simulink model "Testbed_v3"  (R2020a)
settings: Solver=ode23tb  StartTime=0.0  StopTime=20  MaxStep=0.066666666666666671  RelTol=1e-4  EnableMultiTasking=on
undefined symbols (not defined in the file): D11, Delta
libraries: powerlib x95, dspnetwork x75, dspstat3 x52, eePMU x16
(part 2 of 2)

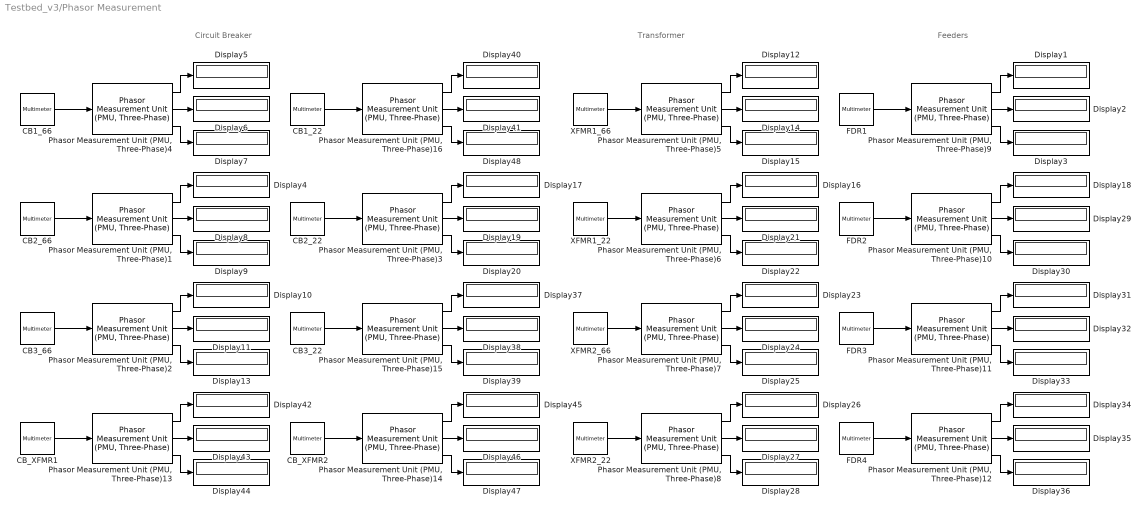
== system Testbed_v3/Phasor Measurement ==
  note: Circuit Breaker
  note: Transformer
  note: Feeders
  CB1_22 : powerlib/Measurements/Multimeter  PhasorSimulation=off  OutputType=Complex  sel=[13 14 15]  L=198  Gain=[1 1 1]  yselected={'Ub: CB1_22KV/Breaker A','Ub: CB1_22KV/Breaker B','Ub: CB1_22KV/Breaker C'};  PSBOutputType=1  PSBequivalent=0  AxesSetting=[0,0.1,-100,100]  Display=0  SavedBlockNames=-11
  CB1_66 : powerlib/Measurements/Multimeter  PhasorSimulation=off  OutputType=Complex  sel=[16 17 18]  L=198  Gain=[1 1 1]  yselected={'Ub: CB1_66KV/Breaker A','Ub: CB1_66KV/Breaker B','Ub: CB1_66KV/Breaker C'};  PSBOutputType=1  PSBequivalent=0  AxesSetting=[0,0.1,-100,100]  Display=0  SavedBlockNames=-11
  CB2_22 : powerlib/Measurements/Multimeter  PhasorSimulation=off  OutputType=Complex  sel=[19 20 21]  L=198  Gain=[1 1 1]  yselected={'Ub: CB2_22KV/Breaker A','Ub: CB2_22KV/Breaker B','Ub: CB2_22KV/Breaker C'};  PSBOutputType=1  PSBequivalent=0  AxesSetting=[0,0.1,-100,100]  Display=0  SavedBlockNames=-11
  CB2_66 : powerlib/Measurements/Multimeter  PhasorSimulation=off  OutputType=Complex  sel=[22 23 24]  L=198  Gain=[1 1 1]  yselected={'Ub: CB2_66KV/Breaker A','Ub: CB2_66KV/Breaker B','Ub: CB2_66KV/Breaker C'};  PSBOutputType=1  PSBequivalent=0  AxesSetting=[0,0.1,-100,100]  Display=0  SavedBlockNames=-11
  CB3_22 : powerlib/Measurements/Multimeter  PhasorSimulation=off  OutputType=Complex  sel=[25 26 27]  L=198  Gain=[1 1 1]  yselected={'Ub: CB3_22KV/Breaker A','Ub: CB3_22KV/Breaker B','Ub: CB3_22KV/Breaker C'};  PSBOutputType=1  PSBequivalent=0  AxesSetting=[0,0.1,-100,100]  Display=0  SavedBlockNames=-11
  CB3_66 : powerlib/Measurements/Multimeter  PhasorSimulation=off  OutputType=Complex  sel=[28 29 30]  L=198  Gain=[1 1 1]  yselected={'Ub: CB3_66KV/Breaker A','Ub: CB3_66KV/Breaker B','Ub: CB3_66KV/Breaker C'};  PSBOutputType=1  PSBequivalent=0  AxesSetting=[0,0.1,-100,100]  Display=0  SavedBlockNames=-11
  CB_XFMR1 : powerlib/Measurements/Multimeter  PhasorSimulation=off  OutputType=Complex  sel=[43 44 45]  L=198  Gain=[1 1 1]  yselected={'Ub: CB_XFMR1/Breaker A','Ub: CB_XFMR1/Breaker B','Ub: CB_XFMR1/Breaker C'};  PSBOutputType=1  PSBequivalent=0  AxesSetting=[0,0.1,-100,100]  Display=0  SavedBlockNames=-11
  CB_XFMR2 : powerlib/Measurements/Multimeter  PhasorSimulation=off  OutputType=Complex  sel=[46 47 48]  L=198  Gain=[1 1 1]  yselected={'Ub: CB_XFMR2/Breaker A','Ub: CB_XFMR2/Breaker B','Ub: CB_XFMR2/Breaker C'};  PSBOutputType=1  PSBequivalent=0  AxesSetting=[0,0.1,-100,100]  Display=0  SavedBlockNames=-11
  Display{1..48} (48 alike) : Display
  FDR1 : powerlib/Measurements/Multimeter  PhasorSimulation=off  OutputType=Complex  sel=[31 32 33]  L=198  Gain=[1 1 1]  yselected={'Ub: CB_FDR1/Breaker A','Ub: CB_FDR1/Breaker B','Ub: CB_FDR1/Breaker C'};  PSBOutputType=1  PSBequivalent=0  AxesSetting=[0,0.1,-100,100]  Display=0  SavedBlockNames=-11
  FDR2 : powerlib/Measurements/Multimeter  PhasorSimulation=off  OutputType=Complex  sel=[34 35 36]  L=198  Gain=[1 1 1]  yselected={'Ub: CB_FDR2/Breaker A','Ub: CB_FDR2/Breaker B','Ub: CB_FDR2/Breaker C'};  PSBOutputType=1  PSBequivalent=0  AxesSetting=[0,0.1,-100,100]  Display=0  SavedBlockNames=-11
  FDR3 : powerlib/Measurements/Multimeter  PhasorSimulation=off  OutputType=Complex  sel=[37 38 39]  L=198  Gain=[1 1 1]  yselected={'Ub: CB_FDR3/Breaker A','Ub: CB_FDR3/Breaker B','Ub: CB_FDR3/Breaker C'};  PSBOutputType=1  PSBequivalent=0  AxesSetting=[0,0.1,-100,100]  Display=0  SavedBlockNames=-11
  FDR4 : powerlib/Measurements/Multimeter  PhasorSimulation=off  OutputType=Complex  sel=[40 41 42]  L=198  Gain=[1 1 1]  yselected={'Ub: CB_FDR4/Breaker A','Ub: CB_FDR4/Breaker B','Ub: CB_FDR4/Breaker C'};  PSBOutputType=1  PSBequivalent=0  AxesSetting=[0,0.1,-100,100]  Display=0  SavedBlockNames=-11
  Phasor Measurement Unit (PMU, Three-Phase){1..16} (16 alike) : eePMU/Phasor Measurement Unit (PMU, Three-Phase)  frequency=50  Nsr=64  k=1
      settings: SourceProductBaseCode=PS
  XFMR1_22 : powerlib/Measurements/Multimeter  PhasorSimulation=off  OutputType=Complex  sel=[82 82 82]  L=198  Gain=[1 1 1]  yselected={'Uab_w2: Three-Phase Transformer 1 (Two Windings)','Uab_w2: Three-Phase Transformer 1 (Two Windings)','Uab_w2: Three-Phase Transformer 1 (Two Windings)'};  PSBOutputType=1  PSBequivalent=0  AxesSetting=[0,0.1,-100,100]  Display=0  SavedBlockNames=-11
  XFMR1_66 : powerlib/Measurements/Multimeter  PhasorSimulation=off  OutputType=Complex  sel=[79 79 79]  L=198  Gain=[1 1 1]  yselected={'Uag_w1: Three-Phase Transformer 1 (Two Windings)','Uag_w1: Three-Phase Transformer 1 (Two Windings)','Uag_w1: Three-Phase Transformer 1 (Two Windings)'};  PSBOutputType=1  PSBequivalent=0  AxesSetting=[0,0.1,-100,100]  Display=0  SavedBlockNames=-11
  XFMR2_22 : powerlib/Measurements/Multimeter  PhasorSimulation=off  OutputType=Complex  sel=[88 88 88]  L=198  Gain=[1 1 1]  yselected={'Uab_w2: Three-Phase Transformer 2 (Two Windings)','Uab_w2: Three-Phase Transformer 2 (Two Windings)','Uab_w2: Three-Phase Transformer 2 (Two Windings)'};  PSBOutputType=1  PSBequivalent=0  AxesSetting=[0,0.1,-100,100]  Display=0  SavedBlockNames=-11
  XFMR2_66 : powerlib/Measurements/Multimeter  PhasorSimulation=off  OutputType=Complex  sel=[85 85 85]  L=198  Gain=[1 1 1]  yselected={'Uag_w1: Three-Phase Transformer 2 (Two Windings)','Uag_w1: Three-Phase Transformer 2 (Two Windings)','Uag_w1: Three-Phase Transformer 2 (Two Windings)'};  PSBOutputType=1  PSBequivalent=0  AxesSetting=[0,0.1,-100,100]  Display=0  SavedBlockNames=-11
  wires:
  CB1_66/1 -> "Phasor Measurement Unit (PMU, Three-Phase)4"/1
  CB2_66/1 -> "Phasor Measurement Unit (PMU, Three-Phase)1"/1
  CB3_66/1 -> "Phasor Measurement Unit (PMU, Three-Phase)2"/1
  XFMR1_22/1 -> "Phasor Measurement Unit (PMU, Three-Phase)6"/1
  XFMR2_66/1 -> "Phasor Measurement Unit (PMU, Three-Phase)7"/1
  CB2_22/1 -> "Phasor Measurement Unit (PMU, Three-Phase)3"/1
  FDR1/1 -> "Phasor Measurement Unit (PMU, Three-Phase)9"/1
  FDR2/1 -> "Phasor Measurement Unit (PMU, Three-Phase)10"/1
  FDR3/1 -> "Phasor Measurement Unit (PMU, Three-Phase)11"/1
  FDR4/1 -> "Phasor Measurement Unit (PMU, Three-Phase)12"/1
  XFMR1_66/1 -> "Phasor Measurement Unit (PMU, Three-Phase)5"/1
  XFMR2_22/1 -> "Phasor Measurement Unit (PMU, Three-Phase)8"/1
  "Phasor Measurement Unit (PMU, Three-Phase)4"/1 -> Display5/1
  "Phasor Measurement Unit (PMU, Three-Phase)4"/2 -> Display6/1
  "Phasor Measurement Unit (PMU, Three-Phase)4"/3 -> Display7/1
  "Phasor Measurement Unit (PMU, Three-Phase)1"/2 -> Display8/1
  "Phasor Measurement Unit (PMU, Three-Phase)1"/3 -> Display9/1
  "Phasor Measurement Unit (PMU, Three-Phase)1"/1 -> Display4/1
  "Phasor Measurement Unit (PMU, Three-Phase)2"/2 -> Display11/1
  "Phasor Measurement Unit (PMU, Three-Phase)2"/3 -> Display13/1
  "Phasor Measurement Unit (PMU, Three-Phase)2"/1 -> Display10/1
  "Phasor Measurement Unit (PMU, Three-Phase)3"/2 -> Display19/1
  "Phasor Measurement Unit (PMU, Three-Phase)3"/3 -> Display20/1
  "Phasor Measurement Unit (PMU, Three-Phase)3"/1 -> Display17/1
  "Phasor Measurement Unit (PMU, Three-Phase)5"/2 -> Display14/1
  "Phasor Measurement Unit (PMU, Three-Phase)5"/3 -> Display15/1
  "Phasor Measurement Unit (PMU, Three-Phase)5"/1 -> Display12/1
  "Phasor Measurement Unit (PMU, Three-Phase)6"/2 -> Display21/1
  "Phasor Measurement Unit (PMU, Three-Phase)6"/3 -> Display22/1
  "Phasor Measurement Unit (PMU, Three-Phase)6"/1 -> Display16/1
  "Phasor Measurement Unit (PMU, Three-Phase)7"/2 -> Display24/1
  "Phasor Measurement Unit (PMU, Three-Phase)7"/3 -> Display25/1
  "Phasor Measurement Unit (PMU, Three-Phase)7"/1 -> Display23/1
  "Phasor Measurement Unit (PMU, Three-Phase)8"/2 -> Display27/1
  "Phasor Measurement Unit (PMU, Three-Phase)8"/3 -> Display28/1
  "Phasor Measurement Unit (PMU, Three-Phase)8"/1 -> Display26/1
  "Phasor Measurement Unit (PMU, Three-Phase)9"/2 -> Display2/1
  "Phasor Measurement Unit (PMU, Three-Phase)9"/3 -> Display3/1
  "Phasor Measurement Unit (PMU, Three-Phase)9"/1 -> Display1/1
  "Phasor Measurement Unit (PMU, Three-Phase)10"/2 -> Display29/1
  "Phasor Measurement Unit (PMU, Three-Phase)10"/3 -> Display30/1
  "Phasor Measurement Unit (PMU, Three-Phase)10"/1 -> Display18/1
  "Phasor Measurement Unit (PMU, Three-Phase)11"/2 -> Display32/1
  "Phasor Measurement Unit (PMU, Three-Phase)11"/3 -> Display33/1
  "Phasor Measurement Unit (PMU, Three-Phase)11"/1 -> Display31/1
  "Phasor Measurement Unit (PMU, Three-Phase)12"/2 -> Display35/1
  "Phasor Measurement Unit (PMU, Three-Phase)12"/3 -> Display36/1
  "Phasor Measurement Unit (PMU, Three-Phase)12"/1 -> Display34/1
  "Phasor Measurement Unit (PMU, Three-Phase)13"/3 -> Display44/1
  "Phasor Measurement Unit (PMU, Three-Phase)13"/2 -> Display43/1
  "Phasor Measurement Unit (PMU, Three-Phase)13"/1 -> Display42/1
  CB_XFMR1/1 -> "Phasor Measurement Unit (PMU, Three-Phase)13"/1
  "Phasor Measurement Unit (PMU, Three-Phase)14"/3 -> Display47/1
  "Phasor Measurement Unit (PMU, Three-Phase)14"/2 -> Display46/1
  "Phasor Measurement Unit (PMU, Three-Phase)14"/1 -> Display45/1
  CB_XFMR2/1 -> "Phasor Measurement Unit (PMU, Three-Phase)14"/1
  CB3_22/1 -> "Phasor Measurement Unit (PMU, Three-Phase)15"/1
  "Phasor Measurement Unit (PMU, Three-Phase)15"/3 -> Display39/1
  "Phasor Measurement Unit (PMU, Three-Phase)15"/1 -> Display37/1
  "Phasor Measurement Unit (PMU, Three-Phase)15"/2 -> Display38/1
  CB1_22/1 -> "Phasor Measurement Unit (PMU, Three-Phase)16"/1
  "Phasor Measurement Unit (PMU, Three-Phase)16"/3 -> Display48/1
  "Phasor Measurement Unit (PMU, Three-Phase)16"/1 -> Display40/1
  "Phasor Measurement Unit (PMU, Three-Phase)16"/2 -> Display41/1

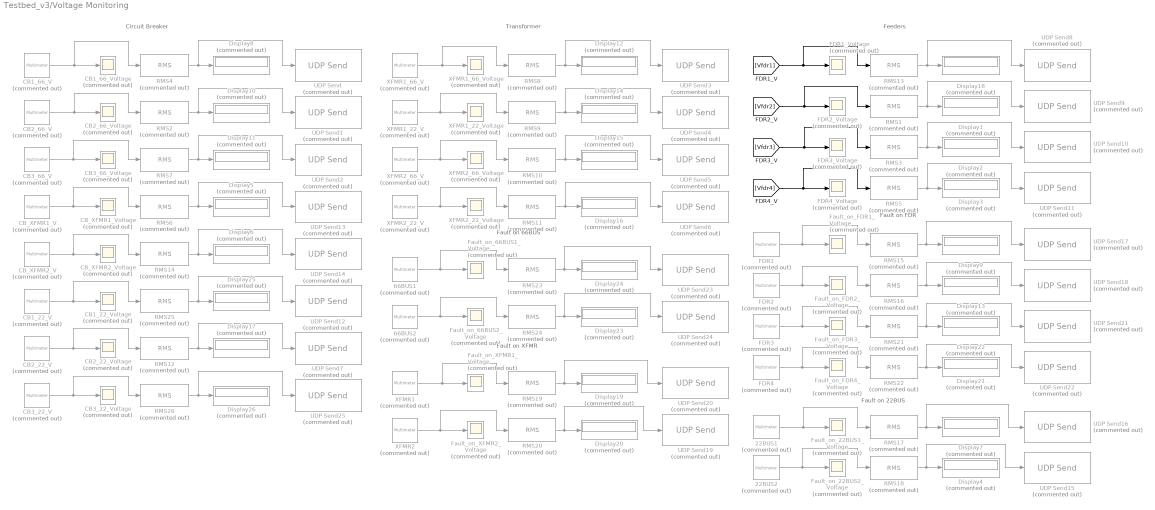
== system Testbed_v3/Voltage Monitoring ==
  note: Circuit Breaker
  note: Transformer
  note: Feeders
  note: Fault on XFMR
  note: Fault on 66BUS
  note: Fault on FDR
  note: Fault on 22BUS
  22BUS1 : powerlib/Measurements/Multimeter  Commented=on  PhasorSimulation=off  OutputType=Complex  sel=[49 50 51]  L=198  Gain=[1 1 1]  yselected={'Ub: Fault_22bus1/Fault A','Ub: Fault_22bus1/Fault B','Ub: Fault_22bus1/Fault C'};  PSBOutputType=1  PSBequivalent=0  AxesSetting=[0,0.1,-100,100]  Display=0  SavedBlockNames=-11
  22BUS2 : powerlib/Measurements/Multimeter  Commented=on  PhasorSimulation=off  OutputType=Complex  sel=[52 53 54]  L=198  Gain=[1 1 1]  yselected={'Ub: Fault_22bus2/Fault A','Ub: Fault_22bus2/Fault B','Ub: Fault_22bus2/Fault C'};  PSBOutputType=1  PSBequivalent=0  AxesSetting=[0,0.1,-100,100]  Display=0  SavedBlockNames=-11
  66BUS1 : powerlib/Measurements/Multimeter  Commented=on  PhasorSimulation=off  OutputType=Complex  sel=[55 56 57]  L=198  Gain=[1 1 1]  yselected={'Ub: Fault_66bus1/Fault A','Ub: Fault_66bus1/Fault B','Ub: Fault_66bus1/Fault C'};  PSBOutputType=1  PSBequivalent=0  AxesSetting=[0,0.1,-100,100]  Display=0  SavedBlockNames=-11
  66BUS2 : powerlib/Measurements/Multimeter  Commented=on  PhasorSimulation=off  OutputType=Complex  sel=[58 59 60]  L=198  Gain=[1 1 1]  yselected={'Ub: Fault_66bus2/Fault A','Ub: Fault_66bus2/Fault B','Ub: Fault_66bus2/Fault C'};  PSBOutputType=1  PSBequivalent=0  AxesSetting=[0,0.1,-100,100]  Display=0  SavedBlockNames=-11
  CB1_22_V : powerlib/Measurements/Multimeter  Commented=on  PhasorSimulation=off  OutputType=Complex  sel=[13 14 15]  L=198  Gain=[1 1 1]  yselected={'Ub: CB1_22KV/Breaker A','Ub: CB1_22KV/Breaker B','Ub: CB1_22KV/Breaker C'};  PSBOutputType=1  PSBequivalent=0  AxesSetting=[0,0.1,-100,100]  Display=0  SavedBlockNames=-11
  CB1_22_Voltage : Scope  Commented=on
  CB1_66_V : powerlib/Measurements/Multimeter  Commented=on  PhasorSimulation=off  OutputType=Complex  sel=[16 17 18]  L=198  Gain=[1 1 1]  yselected={'Ub: CB1_66KV/Breaker A','Ub: CB1_66KV/Breaker B','Ub: CB1_66KV/Breaker C'};  PSBOutputType=1  PSBequivalent=0  AxesSetting=[0,0.1,-100,100]  Display=0  SavedBlockNames=-11
  CB1_66_Voltage : Scope  Commented=on
  CB2_22_V : powerlib/Measurements/Multimeter  Commented=on  PhasorSimulation=off  OutputType=Complex  sel=[19 20 21]  L=198  Gain=[1 1 1]  yselected={'Ub: CB2_22KV/Breaker A','Ub: CB2_22KV/Breaker B','Ub: CB2_22KV/Breaker C'};  PSBOutputType=1  PSBequivalent=0  AxesSetting=[0,0.1,-100,100]  Display=0  SavedBlockNames=-11
  CB2_22_Voltage : Scope  Commented=on
  CB2_66_V : powerlib/Measurements/Multimeter  Commented=on  PhasorSimulation=off  OutputType=Complex  sel=[22 23 24]  L=198  Gain=[1 1 1]  yselected={'Ub: CB2_66KV/Breaker A','Ub: CB2_66KV/Breaker B','Ub: CB2_66KV/Breaker C'};  PSBOutputType=1  PSBequivalent=0  AxesSetting=[0,0.1,-100,100]  Display=0  SavedBlockNames=-11
  CB2_66_Voltage : Scope  Commented=on
  CB3_22_V : powerlib/Measurements/Multimeter  Commented=on  PhasorSimulation=off  OutputType=Complex  sel=[25 26 27]  L=198  Gain=[1 1 1]  yselected={'Ub: CB3_22KV/Breaker A','Ub: CB3_22KV/Breaker B','Ub: CB3_22KV/Breaker C'};  PSBOutputType=1  PSBequivalent=0  AxesSetting=[0,0.1,-100,100]  Display=0  SavedBlockNames=-11
  CB3_22_Voltage : Scope  Commented=on
  CB3_66_V : powerlib/Measurements/Multimeter  Commented=on  PhasorSimulation=off  OutputType=Complex  sel=[28 29 30]  L=198  Gain=[1 1 1]  yselected={'Ub: CB3_66KV/Breaker A','Ub: CB3_66KV/Breaker B','Ub: CB3_66KV/Breaker C'};  PSBOutputType=1  PSBequivalent=0  AxesSetting=[0,0.1,-100,100]  Display=0  SavedBlockNames=-11
  CB3_66_Voltage : Scope  Commented=on
  CB_XFMR1_V : powerlib/Measurements/Multimeter  Commented=on  PhasorSimulation=off  OutputType=Complex  sel=[43 44 45]  L=198  Gain=[1 1 1]  yselected={'Ub: CB_XFMR1/Breaker A','Ub: CB_XFMR1/Breaker B','Ub: CB_XFMR1/Breaker C'};  PSBOutputType=1  PSBequivalent=0  AxesSetting=[0,0.1,-100,100]  Display=0  SavedBlockNames=-11
  CB_XFMR1_Voltage : Scope  Commented=on
  CB_XFMR2_V : powerlib/Measurements/Multimeter  Commented=on  PhasorSimulation=off  OutputType=Complex  sel=[46 47 48]  L=198  Gain=[1 1 1]  yselected={'Ub: CB_XFMR2/Breaker A','Ub: CB_XFMR2/Breaker B','Ub: CB_XFMR2/Breaker C'};  PSBOutputType=1  PSBequivalent=0  AxesSetting=[0,0.1,-100,100]  Display=0  SavedBlockNames=-11
  CB_XFMR2_Voltage : Scope  Commented=on
  Display{1..26} (26 alike) : Display  Commented=on
  FDR1 : powerlib/Measurements/Multimeter  Commented=on  PhasorSimulation=off  OutputType=Complex  sel=[61 62 63]  L=198  Gain=[1 1 1]  yselected={'Ub: Fault_FDR1/Fault A','Ub: Fault_FDR1/Fault B','Ub: Fault_FDR1/Fault C'};  PSBOutputType=1  PSBequivalent=0  AxesSetting=[0,0.1,-100,100]  Display=0  SavedBlockNames=-11
  FDR1_Voltage : Scope  Commented=on
  FDR2 : powerlib/Measurements/Multimeter  Commented=on  PhasorSimulation=off  OutputType=Complex  sel=[64 65 66]  L=198  Gain=[1 1 1]  yselected={'Ub: Fault_FDR2/Fault A','Ub: Fault_FDR2/Fault B','Ub: Fault_FDR2/Fault C'};  PSBOutputType=1  PSBequivalent=0  AxesSetting=[0,0.1,-100,100]  Display=0  SavedBlockNames=-11
  FDR2_Voltage : Scope  Commented=on
  FDR3 : powerlib/Measurements/Multimeter  Commented=on  PhasorSimulation=off  OutputType=Complex  sel=[67 68 69]  L=198  Gain=[1 1 1]  yselected={'Ub: Fault_FDR3/Fault A','Ub: Fault_FDR3/Fault B','Ub: Fault_FDR3/Fault C'};  PSBOutputType=1  PSBequivalent=0  AxesSetting=[0,0.1,-100,100]  Display=0  SavedBlockNames=-11
  FDR3_Voltage : Scope  Commented=on
  FDR4 : powerlib/Measurements/Multimeter  Commented=on  PhasorSimulation=off  OutputType=Complex  sel=[70 71 72]  L=198  Gain=[1 1 1]  yselected={'Ub: Fault_FDR4/Fault A','Ub: Fault_FDR4/Fault B','Ub: Fault_FDR4/Fault C'};  PSBOutputType=1  PSBequivalent=0  AxesSetting=[0,0.1,-100,100]  Display=0  SavedBlockNames=-11
  FDR4_Voltage : Scope  Commented=on
  Fault_on_22BUS1_Voltage : Scope  Commented=on
  Fault_on_22BUS2_Voltage : Scope  Commented=on
  Fault_on_66BUS1_Voltage : Scope  Commented=on
  Fault_on_66BUS2_Voltage : Scope  Commented=on
  Fault_on_FDR1_Voltage : Scope  Commented=on
  Fault_on_FDR2_Voltage : Scope  Commented=on
  Fault_on_FDR3_Voltage : Scope  Commented=on
  Fault_on_FDR4_Voltage : Scope  Commented=on
  Fault_on_XFMR1_Voltage : Scope  Commented=on
  Fault_on_XFMR2_Voltage : Scope  Commented=on
  RMS{1..26} (26 alike) : dspstat3/RMS  Commented=on  run=off  directionMode=Specified dimension  dimension=1  reset_popup=None
  UDP Send : dspnetwork/UDP Send  Commented=on  remoteURL='23.23.23.255'  remotePort=16601  localURL='0.0.0.0'  localPortSource=Automatically determine  localPort=-1  sendBufferSize=8192  sampletime=-1  blockPlatform=[]  separateLengthPort=0
  UDP Send1 : dspnetwork/UDP Send  Commented=on  remoteURL='23.23.23.255'  remotePort=16602  localURL='0.0.0.0'  localPortSource=Automatically determine  localPort=-1  sendBufferSize=8192  sampletime=-1  blockPlatform=[]  separateLengthPort=0
  UDP Send10 : dspnetwork/UDP Send  Commented=on  remoteURL='23.23.23.255'  remotePort=11103  localURL='0.0.0.0'  localPortSource=Automatically determine  localPort=-1  sendBufferSize=8192  sampletime=-1  blockPlatform=[]  separateLengthPort=0
  UDP Send11 : dspnetwork/UDP Send  Commented=on  remoteURL='23.23.23.255'  remotePort=11104  localURL='0.0.0.0'  localPortSource=Automatically determine  localPort=-1  sendBufferSize=8192  sampletime=-1  blockPlatform=[]  separateLengthPort=0
  UDP Send12 : dspnetwork/UDP Send  Commented=on  remoteURL='23.23.23.255'  remotePort=12201  localURL='0.0.0.0'  localPortSource=Automatically determine  localPort=-1  sendBufferSize=8192  sampletime=-1  blockPlatform=[]  separateLengthPort=0
  UDP Send13 : dspnetwork/UDP Send  Commented=on  remoteURL='23.23.23.255'  remotePort=13301  localURL='0.0.0.0'  localPortSource=Automatically determine  localPort=-1  sendBufferSize=8192  sampletime=-1  blockPlatform=[]  separateLengthPort=0
  UDP Send14 : dspnetwork/UDP Send  Commented=on  remoteURL='23.23.23.255'  remotePort=13302  localURL='0.0.0.0'  localPortSource=Automatically determine  localPort=-1  sendBufferSize=8192  sampletime=-1  blockPlatform=[]  separateLengthPort=0
  UDP Send15 : dspnetwork/UDP Send  Commented=on  remoteURL='23.23.23.255'  remotePort=12232  localURL='0.0.0.0'  localPortSource=Automatically determine  localPort=-1  sendBufferSize=8192  sampletime=-1  blockPlatform=[]  separateLengthPort=0
  UDP Send16 : dspnetwork/UDP Send  Commented=on  remoteURL='23.23.23.255'  remotePort=12231  localURL='0.0.0.0'  localPortSource=Automatically determine  localPort=-1  sendBufferSize=8192  sampletime=-1  blockPlatform=[]  separateLengthPort=0
  UDP Send17 : dspnetwork/UDP Send  Commented=on  remoteURL='23.23.23.255'  remotePort=11131  localURL='0.0.0.0'  localPortSource=Automatically determine  localPort=-1  sendBufferSize=8192  sampletime=-1  blockPlatform=[]  separateLengthPort=0
  UDP Send18 : dspnetwork/UDP Send  Commented=on  remoteURL='23.23.23.255'  remotePort=11132  localURL='0.0.0.0'  localPortSource=Automatically determine  localPort=-1  sendBufferSize=8192  sampletime=-1  blockPlatform=[]  separateLengthPort=0
  UDP Send19 : dspnetwork/UDP Send  Commented=on  remoteURL='23.23.23.255'  remotePort=13332  localURL='0.0.0.0'  localPortSource=Automatically determine  localPort=-1  sendBufferSize=8192  sampletime=-1  blockPlatform=[]  separateLengthPort=0
  UDP Send2 : dspnetwork/UDP Send  Commented=on  remoteURL='23.23.23.255'  remotePort=16603  localURL='0.0.0.0'  localPortSource=Automatically determine  localPort=-1  sendBufferSize=8192  sampletime=-1  blockPlatform=[]  separateLengthPort=0
  UDP Send20 : dspnetwork/UDP Send  Commented=on  remoteURL='23.23.23.255'  remotePort=13331  localURL='0.0.0.0'  localPortSource=Automatically determine  localPort=-1  sendBufferSize=8192  sampletime=-1  blockPlatform=[]  separateLengthPort=0
  UDP Send21 : dspnetwork/UDP Send  Commented=on  remoteURL='23.23.23.255'  remotePort=11133  localURL='0.0.0.0'  localPortSource=Automatically determine  localPort=-1  sendBufferSize=8192  sampletime=-1  blockPlatform=[]  separateLengthPort=0
  UDP Send22 : dspnetwork/UDP Send  Commented=on  remoteURL='23.23.23.255'  remotePort=11134  localURL='0.0.0.0'  localPortSource=Automatically determine  localPort=-1  sendBufferSize=8192  sampletime=-1  blockPlatform=[]  separateLengthPort=0
  UDP Send23 : dspnetwork/UDP Send  Commented=on  remoteURL='23.23.23.255'  remotePort=16631  localURL='0.0.0.0'  localPortSource=Automatically determine  localPort=-1  sendBufferSize=8192  sampletime=-1  blockPlatform=[]  separateLengthPort=0
  UDP Send24 : dspnetwork/UDP Send  Commented=on  remoteURL='23.23.23.255'  remotePort=16632  localURL='0.0.0.0'  localPortSource=Automatically determine  localPort=-1  sendBufferSize=8192  sampletime=-1  blockPlatform=[]  separateLengthPort=0
  UDP Send25 : dspnetwork/UDP Send  Commented=on  remoteURL='23.23.23.255'  remotePort=12203  localURL='0.0.0.0'  localPortSource=Automatically determine  localPort=-1  sendBufferSize=8192  sampletime=-1  blockPlatform=[]  separateLengthPort=0
  UDP Send3 : dspnetwork/UDP Send  Commented=on  remoteURL='23.23.23.255'  remotePort=15501  localURL='0.0.0.0'  localPortSource=Automatically determine  localPort=-1  sendBufferSize=8192  sampletime=-1  blockPlatform=[]  separateLengthPort=0
  UDP Send4 : dspnetwork/UDP Send  Commented=on  remoteURL='23.23.23.255'  remotePort=14401  localURL='0.0.0.0'  localPortSource=Automatically determine  localPort=-1  sendBufferSize=8192  sampletime=-1  blockPlatform=[]  separateLengthPort=0
  UDP Send5 : dspnetwork/UDP Send  Commented=on  remoteURL='23.23.23.255'  remotePort=15502  localURL='0.0.0.0'  localPortSource=Automatically determine  localPort=-1  sendBufferSize=8192  sampletime=-1  blockPlatform=[]  separateLengthPort=0
  UDP Send6 : dspnetwork/UDP Send  Commented=on  remoteURL='23.23.23.255'  remotePort=14402  localURL='0.0.0.0'  localPortSource=Automatically determine  localPort=-1  sendBufferSize=8192  sampletime=-1  blockPlatform=[]  separateLengthPort=0
  UDP Send7 : dspnetwork/UDP Send  Commented=on  remoteURL='23.23.23.255'  remotePort=12202  localURL='0.0.0.0'  localPortSource=Automatically determine  localPort=-1  sendBufferSize=8192  sampletime=-1  blockPlatform=[]  separateLengthPort=0
  UDP Send8 : dspnetwork/UDP Send  Commented=on  remoteURL='23.23.23.255'  remotePort=11101  localURL='0.0.0.0'  localPortSource=Automatically determine  localPort=-1  sendBufferSize=8192  sampletime=-1  blockPlatform=[]  separateLengthPort=0
  UDP Send9 : dspnetwork/UDP Send  Commented=on  remoteURL='23.23.23.255'  remotePort=11102  localURL='0.0.0.0'  localPortSource=Automatically determine  localPort=-1  sendBufferSize=8192  sampletime=-1  blockPlatform=[]  separateLengthPort=0
  XFMR1 : powerlib/Measurements/Multimeter  Commented=on  PhasorSimulation=off  OutputType=Complex  sel=[73 74 75]  L=198  Gain=[1 1 1]  yselected={'Ub: Fault_XFMR1/Fault A','Ub: Fault_XFMR1/Fault B','Ub: Fault_XFMR1/Fault C'};  PSBOutputType=1  PSBequivalent=0  AxesSetting=[0,0.1,-100,100]  Display=0  SavedBlockNames=-11
  XFMR1_22_V : powerlib/Measurements/Multimeter  Commented=on  PhasorSimulation=off  OutputType=Complex  sel=[82 83 84]  L=198  Gain=[1 1 1]  yselected={'Uab_w2: Three-Phase Transformer 1 (Two Windings)','Ubc_w2: Three-Phase Transformer 1 (Two Windings)','Uca_w2: Three-Phase Transformer 1 (Two Windings)'};  PSBOutputType=1  PSBequivalent=0  AxesSetting=[0,0.1,-100,100]  Display=0  SavedBlockNames=-11
  XFMR1_22_Voltage : Scope  Commented=on
  XFMR1_66_V : powerlib/Measurements/Multimeter  Commented=on  PhasorSimulation=off  OutputType=Complex  sel=[79 80 81]  L=198  Gain=[1 1 1]  yselected={'Uag_w1: Three-Phase Transformer 1 (Two Windings)','Ubg_w1: Three-Phase Transformer 1 (Two Windings)','Ucg_w1: Three-Phase Transformer 1 (Two Windings)'};  PSBOutputType=1  PSBequivalent=0  AxesSetting=[0,0.1,-100,100]  Display=0  SavedBlockNames=-11
  XFMR1_66_Voltage : Scope  Commented=on
  XFMR2 : powerlib/Measurements/Multimeter  Commented=on  PhasorSimulation=off  OutputType=Complex  sel=[76 77 78]  L=198  Gain=[1 1 1]  yselected={'Ub: Fault_XFMR2/Fault A','Ub: Fault_XFMR2/Fault B','Ub: Fault_XFMR2/Fault C'};  PSBOutputType=1  PSBequivalent=0  AxesSetting=[0,0.1,-100,100]  Display=0  SavedBlockNames=-11
  XFMR2_22_V : powerlib/Measurements/Multimeter  Commented=on  PhasorSimulation=off  OutputType=Complex  sel=[88 89 90]  L=198  Gain=[1 1 1]  yselected={'Uab_w2: Three-Phase Transformer 2 (Two Windings)','Ubc_w2: Three-Phase Transformer 2 (Two Windings)','Uca_w2: Three-Phase Transformer 2 (Two Windings)'};  PSBOutputType=1  PSBequivalent=0  AxesSetting=[0,0.1,-100,100]  Display=0  SavedBlockNames=-11
  XFMR2_22_Voltage : Scope  Commented=on
  XFMR2_66_V : powerlib/Measurements/Multimeter  Commented=on  PhasorSimulation=off  OutputType=Complex  sel=[85 86 87]  L=198  Gain=[1 1 1]  yselected={'Uag_w1: Three-Phase Transformer 2 (Two Windings)','Ubg_w1: Three-Phase Transformer 2 (Two Windings)','Ucg_w1: Three-Phase Transformer 2 (Two Windings)'};  PSBOutputType=1  PSBequivalent=0  AxesSetting=[0,0.1,-100,100]  Display=0  SavedBlockNames=-11
  XFMR2_66_Voltage : Scope  Commented=on
  wires:
  CB1_66_V/1 -> RMS4/1, CB1_66_Voltage/1
  RMS4/1 -> UDP Send/1, Display8/1
  RMS2/1 -> UDP Send1/1, Display10/1
  CB2_66_V/1 -> RMS2/1, CB2_66_Voltage/1
  CB3_66_V/1 -> RMS7/1, CB3_66_Voltage/1
  RMS7/1 -> UDP Send2/1, Display11/1
  RMS8/1 -> UDP Send3/1, Display12/1
  XFMR1_22_V/1 -> RMS9/1, XFMR1_22_Voltage/1
  RMS9/1 -> UDP Send4/1, Display14/1
  XFMR2_66_V/1 -> RMS10/1, XFMR2_66_Voltage/1
  RMS10/1 -> UDP Send5/1, Display15/1
  RMS11/1 -> UDP Send6/1, Display16/1
  [Vfdr1] -> RMS13/1, FDR1_Voltage/1
  RMS13/1 -> UDP Send8/1, Display18/1
  RMS1/1 -> UDP Send9/1, Display1/1
  [Vfdr2] -> RMS1/1, FDR2_Voltage/1
  RMS3/1 -> UDP Send10/1, Display2/1
  [Vfdr3] -> RMS3/1, FDR3_Voltage/1
  RMS5/1 -> UDP Send11/1, Display3/1
  [Vfdr4] -> RMS5/1, FDR4_Voltage/1
  XFMR1_66_V/1 -> RMS8/1, XFMR1_66_Voltage/1
  XFMR2_22_V/1 -> RMS11/1, XFMR2_22_Voltage/1
  CB_XFMR2_V/1 -> RMS14/1, CB_XFMR2_Voltage/1
  RMS14/1 -> UDP Send14/1, Display6/1
  CB_XFMR1_V/1 -> RMS6/1, CB_XFMR1_Voltage/1
  RMS6/1 -> UDP Send13/1, Display5/1
  RMS16/1 -> UDP Send18/1, Display13/1
  XFMR1/1 -> RMS19/1, Fault_on_XFMR1_Voltage/1
  RMS15/1 -> UDP Send17/1, Display9/1
  FDR1/1 -> RMS15/1, Fault_on_FDR1_Voltage/1
  XFMR2/1 -> RMS20/1, Fault_on_XFMR2_Voltage/1
  RMS21/1 -> UDP Send21/1, Display22/1
  FDR2/1 -> RMS16/1, Fault_on_FDR2_Voltage/1
  66BUS2/1 -> RMS24/1, Fault_on_66BUS2_Voltage/1
  22BUS1/1 -> RMS17/1, Fault_on_22BUS1_Voltage/1
  66BUS1/1 -> RMS23/1, Fault_on_66BUS1_Voltage/1
  RMS23/1 -> UDP Send23/1, Display24/1
  RMS22/1 -> UDP Send22/1, Display21/1
  RMS20/1 -> UDP Send19/1, Display20/1
  22BUS2/1 -> RMS18/1, Fault_on_22BUS2_Voltage/1
  RMS17/1 -> UDP Send16/1, Display7/1
  RMS18/1 -> UDP Send15/1, Display4/1
  RMS24/1 -> UDP Send24/1, Display23/1
  FDR3/1 -> RMS21/1, Fault_on_FDR3_Voltage/1
  RMS19/1 -> UDP Send20/1, Display19/1
  FDR4/1 -> RMS22/1, Fault_on_FDR4_Voltage/1
  CB2_22_V/1 -> RMS12/1, CB2_22_Voltage/1
  RMS12/1 -> UDP Send7/1, Display17/1
  CB1_22_V/1 -> RMS25/1, CB1_22_Voltage/1
  RMS25/1 -> UDP Send12/1, Display25/1
  CB3_22_V/1 -> RMS26/1, CB3_22_Voltage/1
  RMS26/1 -> UDP Send25/1, Display26/1

== matlab function Testbed_v3/UTC Time Record ==
  data: time output
function time  = fcn

   eml.extrinsic('datetime');
   eml.extrinsic('posixtime');


   time = 0;

   [time] = posixtime(datetime('now', 'TimeZone','local'));
end
